simulink model "differentcontroller"  (R2018a)
settings: Solver=FixedStepAuto  StartTime=0.0  StopTime=10  FixedStep=0.001  MaxStep=0.005  MinStep=0.001  RelTol=1e-3
libraries: simulink x6
settings Model: Creator=Dell  LastModifiedBy=Dell
settings SolverCC: InitialStep=0.001

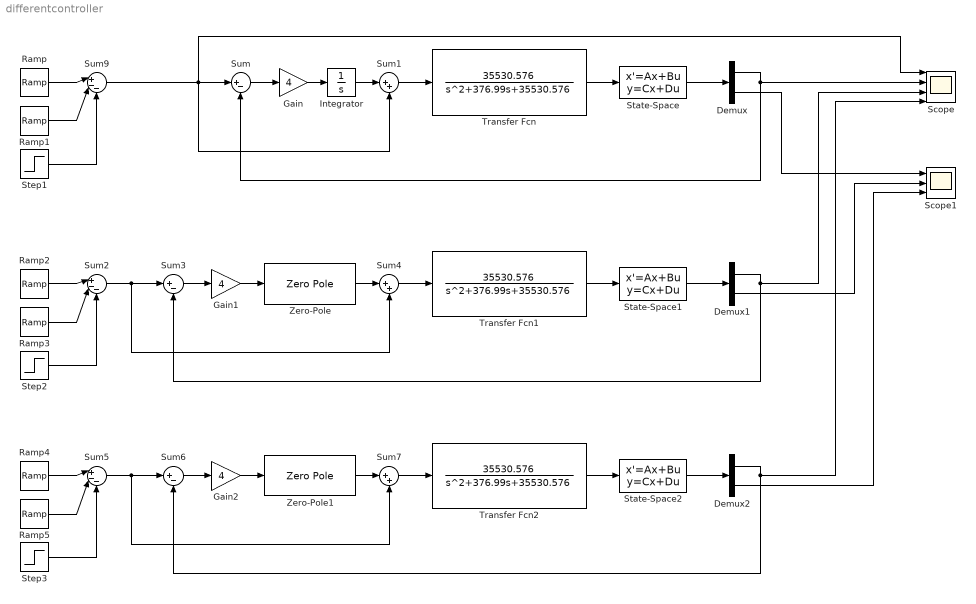
== system differentcontroller ==
  Demux : Demux  Outputs=2
  Demux1 : Demux  Outputs=2
  Demux2 : Demux  Outputs=2
  Gain : Gain  Gain=4
  Gain1 : Gain  Gain=4
  Gain2 : Gain  Gain=4
  Integrator : Integrator
  Ramp : simulink/Sources/Ramp  slope=150  start=1  InitialOutput=0
  Ramp1 : simulink/Sources/Ramp  slope=150  start=1.1  InitialOutput=0
  Ramp2 : simulink/Sources/Ramp  slope=150  start=1  InitialOutput=0
  Ramp3 : simulink/Sources/Ramp  slope=150  start=1.1  InitialOutput=0
  Ramp4 : simulink/Sources/Ramp  slope=150  start=1  InitialOutput=0
  Ramp5 : simulink/Sources/Ramp  slope=150  start=1.1  InitialOutput=0
  Scope : Scope  NumInputPorts=4
  Scope1 : Scope  NumInputPorts=3
  State-Space : StateSpace  A=-5.443  B=5.063  C=[0.4557;-108.86]  D=[0.5063;101.266]  InitialCondition=0
  State-Space1 : StateSpace  A=-5.443  B=5.063  C=[0.4557;-108.86]  D=[0.5063;101.266]  InitialCondition=0
  State-Space2 : StateSpace  A=-5.443  B=5.063  C=[0.4557;-108.86]  D=[0.5063;101.266]  InitialCondition=0
  Step1 : Step  Time=5  After=15  SampleTime=0
  Step2 : Step  Time=5  After=15  SampleTime=0
  Step3 : Step  Time=5  After=15  SampleTime=0
  Sum : Sum  Inputs=|+-
  Sum1 : Sum  Inputs=|++
  Sum2 : Sum  Inputs=|+--
  Sum3 : Sum  Inputs=|+-
  Sum4 : Sum  Inputs=|++
  Sum5 : Sum  Inputs=|+--
  Sum6 : Sum  Inputs=|+-
  Sum7 : Sum  Inputs=|++
  Sum9 : Sum  Inputs=|+--
  Transfer Fcn : TransferFcn  Numerator=[35530.576]  Denominator=[1 376.99 35530.576]
  Transfer Fcn1 : TransferFcn  Numerator=[35530.576]  Denominator=[1 376.99 35530.576]
  Transfer Fcn2 : TransferFcn  Numerator=[35530.576]  Denominator=[1 376.99 35530.576]
  Zero-Pole : ZeroPole  Zeros=[-2.5]  Poles=[0]
  Zero-Pole1 : ZeroPole  Zeros=[-2.5]  Poles=[-0.1]
  wires:
  Sum2/1 -> Sum4/2, Sum3/1
  Sum5/1 -> Sum7/2, Sum6/1
  Ramp3/1 -> Sum2/2
  Ramp4/1 -> Sum5/1
  Zero-Pole1/1 -> Sum7/1
  Gain2/1 -> Zero-Pole1/1
  Step3/1 -> Sum5/3
  Ramp5/1 -> Sum5/2
  Transfer Fcn1/1 -> State-Space1/1
  Sum6/1 -> Gain2/1
  Sum1/1 -> Transfer Fcn/1
  State-Space2/1 -> Demux2/1
  Demux2/2 -> Scope1/3
  State-Space1/1 -> Demux1/1
  Sum7/1 -> Transfer Fcn2/1
  Ramp2/1 -> Sum2/1
  Gain/1 -> Integrator/1
  Step1/1 -> Sum9/3
  Demux1/1 -> Scope/3, Sum3/2
  Sum/1 -> Gain/1
  Demux/2 -> Scope1/1
  Zero-Pole/1 -> Sum4/1
  Gain1/1 -> Zero-Pole/1
  Demux2/1 -> Scope/4, Sum6/2
  Demux1/2 -> Scope1/2
  Transfer Fcn/1 -> State-Space/1
  Sum4/1 -> Transfer Fcn1/1
  Integrator/1 -> Sum1/1
  Step2/1 -> Sum2/3
  Transfer Fcn2/1 -> State-Space2/1
  Ramp/1 -> Sum9/1
  State-Space/1 -> Demux/1
  Ramp1/1 -> Sum9/2
  Sum9/1 -> Scope/1, Sum1/2, Sum/1
  Sum3/1 -> Gain1/1
  Demux/1 -> Scope/2, Sum/2
